simulink model "RefModel_TaskOutput"  (R2015b)
settings: configuration reference "CenterOutReachConfigSet" (kept outside this file)
undefined symbols (not defined in the file or in its folder): SimulinkParameter_TunableNote
settings Model: Creator=djoshea  LastModifiedBy=shenoylab
settings ConfigSetRef: SourceLocation=Base Workspace

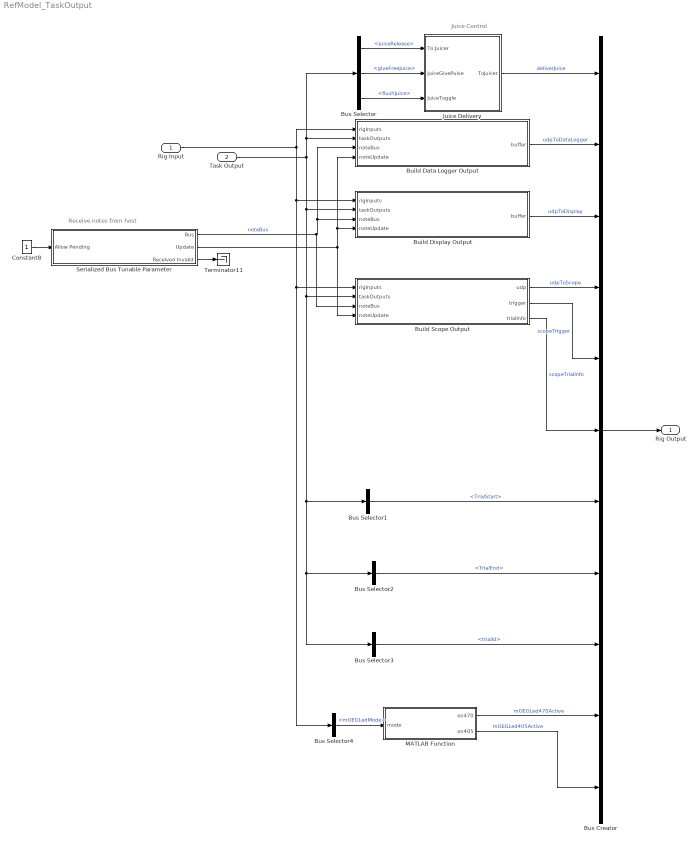
== system RefModel_TaskOutput ==
  note: Juice Control
  note: Receive notes from host
  Rig Input : Inport  OutDataTypeStr=Bus: RigInputBus  PortDimensions=1  SampleTime=[0.001,0]  Interpolate=off  BusOutputAsStruct=on
  Task Output : Inport  Port=2  OutDataTypeStr=Bus: TaskOutputBus  PortDimensions=1  SampleTime=[0.001,0]  Interpolate=off  BusOutputAsStruct=on
  Build Data Logger Output : MATLAB Function  TreatAsAtomicUnit=on
  Build Display Output : MATLAB Function  TreatAsAtomicUnit=on
  Build Scope Output : MATLAB Function  TreatAsAtomicUnit=on
  Bus Creator : BusCreator  Inputs=11  OutDataTypeStr=Bus: RigOutputBus  NonVirtualBus=on
  Bus Selector : BusSelector  OutputSignals=juiceRelease,taskControl.giveFreeJuice,taskControl.flushJuice
  Bus Selector1 : BusSelector  OutputSignals=TrialStart
  Bus Selector2 : BusSelector  OutputSignals=TrialEnd
  Bus Selector3 : BusSelector  OutputSignals=trialId
  Bus Selector4 : BusSelector  OutputSignals=scopeState.mOEGLedMode
  Constant8 : Constant  OutDataTypeStr=uint8
  Juice Delivery : Subsystem
  MATLAB Function : MATLAB Function  TreatAsAtomicUnit=on
  Serialized Bus Tunable Parameter : Subsystem  AncestorBlock=libBusSerialize/Serialized Bus Tunable Parameter  mask(BusSerialize Tunable Parameter Block){paramName='TunableNote'}
      mask prompts: paramName "Parameter Name"
      mask help: This block provides the value of a tunable Simulink.Parameter into the model. Since tunable parameters with xPC target can only be doubles, the functions BusSerialize.createTunableParameter and BusSerialize.setTunableParameter automatically handle typecasting and update counter insertion, and this block handles update detection, typecasting, and reshaping back to the original form. Currently, variable size parameters are not supported.
      mask init:
      | BusSerialize.maskSerializedBusTunableParameterBlockUpdate(gcb);
      mask Display:
      | port_label('output', 1, paramName);
      | port_label('output', 2, 'Update');
      | port_label('output', 3, 'Received Invalid');
      | port_label('input', 1, 'Allow Pending');
  Terminator11 : Terminator
  Rig Output : Outport  OutDataTypeStr=Bus: RigOutputBus  PortDimensions=1  SampleTime=[0.001,0]  BusOutputAsStruct=on
  wires:
  Rig Input/1 -> Bus Selector4/1, Build Scope Output/1(rigInputs), Build Display Output/1(rigInputs), Build Data Logger Output/1(rigInputs)
  Bus Creator/1 -> Rig Output/1
  Build Data Logger Output/1(buffer) -> Bus Creator/2  "udpToDataLogger"
  Build Display Output/1(buffer) -> Bus Creator/3  "udpToDisplay"
  Bus Selector/2 -> Juice Delivery/2(JuiceGivePulse)  "<giveFreeJuice>"
  Bus Selector/1 -> Juice Delivery/1(To Juicer)  "<juiceRelease>"
  Bus Selector/3 -> Juice Delivery/3(JuiceToggle)  "<flushJuice>"
  Juice Delivery/1(ToJuicer) -> Bus Creator/1  "deliverJuice"
  Constant8/1 -> Serialized Bus Tunable Parameter/1(Allow Pending)
  Serialized Bus Tunable Parameter/3(Received Invalid) -> Terminator11/1
  Serialized Bus Tunable Parameter/1(Bus) -> Build Scope Output/3(noteBus), Build Data Logger Output/3(noteBus), Build Display Output/3(noteBus)  "noteBus"
  Bus Selector1/1 -> Bus Creator/7  "<TrialStart>"
  Serialized Bus Tunable Parameter/2(Update) -> Build Scope Output/4(noteUpdate), Build Data Logger Output/4(noteUpdate), Build Display Output/4(noteUpdate)
  Build Scope Output/1(udp) -> Bus Creator/4  "udpToScope"
  Build Scope Output/2(trigger) -> Bus Creator/5  "scopeTrigger"
  Bus Selector2/1 -> Bus Creator/8  "<TrialEnd>"
  Build Scope Output/3(trialInfo) -> Bus Creator/6  "scopeTrialInfo"
  Task Output/1 -> Build Data Logger Output/2(taskOutputs), Bus Selector/1, Bus Selector3/1, Bus Selector2/1, Bus Selector1/1, Build Scope Output/2(taskOutputs), Build Display Output/2(taskOutputs)
  Bus Selector3/1 -> Bus Creator/9  "<trialId>"
  Bus Selector4/1 -> MATLAB Function/1(mode)  "<mOEGLedMode>"
  MATLAB Function/2(on405) -> Bus Creator/11  "mOEGLed405Active"
  MATLAB Function/1(on470) -> Bus Creator/10  "mOEGLed470Active"

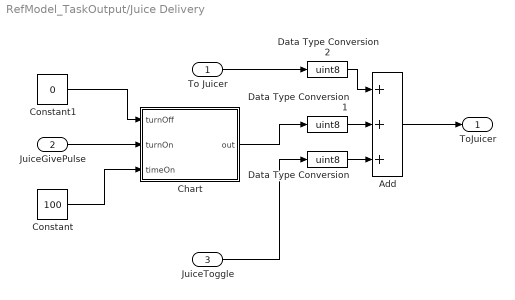
== system RefModel_TaskOutput/Juice Delivery ==
  To Juicer : Inport
  JuiceGivePulse : Inport  Port=2
  JuiceToggle : Inport  Port=3
  Add : Sum  Inputs=+++
  Chart : Stateflow chart  TreatAsAtomicUnit=on
  Constant : Constant  Value=100  OutDataTypeStr=uint32
  Constant1 : Constant  Value=0  OutDataTypeStr=uint8
  Data Type Conversion : DataTypeConversion  OutDataTypeStr=uint8
  Data Type Conversion1 : DataTypeConversion  OutDataTypeStr=uint8
  Data Type Conversion2 : DataTypeConversion  OutDataTypeStr=uint8
  ToJuicer : Outport
  wires:
  Data Type Conversion2/1 -> Add/1
  Data Type Conversion1/1 -> Add/2
  Data Type Conversion/1 -> Add/3
  Constant1/1 -> Chart/1(turnOff)
  JuiceToggle/1 -> Data Type Conversion/1
  Add/1 -> ToJuicer/1
  Constant/1 -> Chart/3(timeOn)
  JuiceGivePulse/1 -> Chart/2(turnOn)
  Chart/1(out) -> Data Type Conversion1/1
  To Juicer/1 -> Data Type Conversion2/1

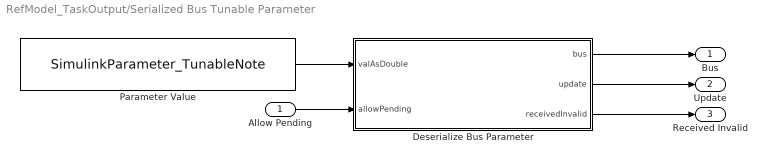
== system RefModel_TaskOutput/Serialized Bus Tunable Parameter ==
  Allow Pending : Inport
  Deserialize Bus Parameter : MATLAB Function  TreatAsAtomicUnit=on
  Parameter Value : Constant  Value=SimulinkParameter_TunableNote  OutDataTypeStr=double
  Bus : Outport  PortDimensions=1
  Update : Outport  Port=2  OutDataTypeStr=uint8  PortDimensions=1
  Received Invalid : Outport  Port=3  OutDataTypeStr=uint8  PortDimensions=1
  wires:
  Parameter Value/1 -> Deserialize Bus Parameter/1(valAsDouble)
  Allow Pending/1 -> Deserialize Bus Parameter/2(allowPending)
  Deserialize Bus Parameter/3(receivedInvalid) -> Received Invalid/1
  Deserialize Bus Parameter/1(bus) -> Bus/1
  Deserialize Bus Parameter/2(update) -> Update/1

== matlab function RefModel_TaskOutput/Build Scope Output ==
  data: udp output uint8 size=RigInfo.outputSizes.udpToScope; rigInputs input Bus: RigInputBus size=1; taskOutputs input Bus: TaskOutputBus size=1; noteBus input Bus: NoteBus size=1; noteUpdate input uint8 size=1; RigInfo parameter size=1; trigger output uint8 size=1; trialInfo output uint8 size=RigInfo.outputSizes.trialInfoToScope
function [udp, trigger, trialInfo] = buildScopeOutput(rigInputs, taskOutputs, noteBus, noteUpdate, RigInfo)
%#codegen

    coder.cinclude('<stdlib.h>'); % for sprintf

    coder.varsize('udp', RigInfo.outputSizes.udpToScope);
    coder.varsize('trialInfo', RigInfo.outputSizes.trialInfoToScope);
    
    bEmpty = zeros(0, 1, 'uint8');
    
    
    

    %initialize persistant variables
    persistent pTrialId;
    if isempty(pTrialId)
        pTrialId = uint32(0);
    end
    
    persistent pConditionId;
    if isempty(pConditionId)
        pConditionId = uint16(0);
    end
    
    persistent pConditionsToDecode;
    if isempty(pConditionsToDecode)
        pConditionsToDecode = uint8(zeros(4,1));
    end
    
    persistent pUseNextFrame;
    if isempty(pUseNextFrame)
        pUseNextFrame = uint8(0);
    end
    
    persistent pImageDecoderTraining;
    if isempty(pImageDecoderTraining)
        pImageDecoderTraining = uint8(0);
    end
    
    persistent pResetDecoder;
    if isempty(pResetDecoder)
        pResetDecoder = uint8(0);
    end
    
    persistent pSaveTag;
    if isempty(pSaveTag)
        pSaveTag = uint32(0);
    end
    
    % detect if any of these have changed and update persistent variable
    doBytePack = false;
    if (taskOutputs.trialId ~= pTrialId)    
        doBytePack = true;
        pTrialId = uint32(taskOutputs.trialId);
    end
    
    if (taskOutputs.condition.conditionId ~= pConditionId)
        doBytePack = true;
        pConditionId = uint16(taskOutputs.condition.conditionId);
    end
    
    if all(taskOutputs.param.conditionsToDecode ~= pConditionsToDecode)
        doBytePack = true;
        pConditionsToDecode = uint8(taskOutputs.param.conditionsToDecode);
    end
    
    if (taskOutputs.trialData.useNextFrame ~= pUseNextFrame)
        doBytePack = true;
        pUseNextFrame = uint8(taskOutputs.trialData.useNextFrame);
    end
    
    if (taskOutputs.param.imageDecoderTraining ~= pImageDecoderTraining)
        doBytePack = true;
        pImageDecoderTraining = uint8(taskOutputs.param.imageDecoderTraining);
    end
    
    if (taskOutputs.param.resetImageDecoder ~= pResetDecoder)
        doBytePack = true;
        pResetDecoder = uint8(taskOutputs.param.resetImageDecoder);
    end
    
    if (taskOutputs.dataLoggerInfo.saveTag ~= pSaveTag)
        doBytePack = true;
        pSaveTag = uint32(taskOutputs.dataLoggerInfo.saveTag);
    end
    
    % Do the byte packing if anything has updated
    if doBytePack
        bHeader = uint8('#D')';
        bTrialId = typecast(taskOutputs.trialId,'uint8')';
        bConditionId = typecast(taskOutputs.condition.conditionId,'uint8')';
        bConditionsToDecode = uint8(taskOutputs.param.conditionsToDecode);  % already a logical
        bUseNextFrame = typecast(taskOutputs.trialData.useNextFrame,'uint8')';
        bImageDecoderTraining = typecast(taskOutputs.param.imageDecoderTraining,'uint8')';
        bResetDecoder = typecast(taskOutputs.param.resetImageDecoder,'uint8')';
        bSaveTag = typecast(pSaveTag, 'uint8')';
        udp = [bHeader; bTrialId; bConditionId; bConditionsToDecode; ...
            bUseNextFrame; bImageDecoderTraining; bResetDecoder; bSaveTag];
        trigger = uint8(1);
    else
        trigger = uint8(0);
        udp = bEmpty;
    end
    
    if ~isempty(udp)
        % add null-terminator for udp and make sure byte count is even,
        % needed for Windows, not sure why
        if mod(numel(udp), 2) == 0
            udp = [udp; uint8(' '); uint8(0)];
        else
            udp = [udp; uint8(0)];
        end
    end
    
     maxNextTrial = 500;
     trialInfo = bEmpty;

    % serialize scope commands
    if taskOutputs.taskControl.controlImaging && ~isempty(taskOutputs.scopeCommandQueue)
        % loop through scope commands and generate the command text for
        % each 
        coder.varsize('bNextTrial', maxNextTrial);
        for i = 1:numel(taskOutputs.scopeCommandQueue)
            command = taskOutputs.scopeCommandQueue(i);
            
            switch command
                case ScopeCommand.NextTrial
                   % also generate a command to send to the PrairieView
                    % voltage recording
                    nBytes = int32(0);
                    trialInfoBuffer = zeros(RigInfo.outputSizes.trialInfoToScope, 1, 'uint8');
                    nBytes = coder.ceval('sprintf', coder.ref(trialInfoBuffer), ...
                        ['id=%d,c=%d,d=' enumToString_DirectionName(taskOutputs.condition.targetDirectionName)' ';' uint8(0)], ...
                        taskOutputs.trialId, taskOutputs.condition.conditionId);
                     if nBytes > RigInfo.outputSizes.trialInfoToScope
                         trialInfo = trialInfoBuffer(1:RigInfo.outputSizes.trialInfoToScope);
                     else
                         trialInfo = trialInfoBuffer(1:nBytes);
                     end
            end
        end
    end
    
    
    
    
end

== matlab function RefModel_TaskOutput/MATLAB Function ==
  data: mode input Enum: LedMode size=1; on470 output uint8 size=1; on405 output uint8 size=1
function [on470, on405] = getLedStatus(mode)
%#codegen

    on470 = uint8(0);
    on405 = uint8(0);
    
    switch mode
        case LedMode.Off
            
        case LedMode.CW405
            on405 = uint8(1);

        case LedMode.CW470
            on470 = uint8(1);
    
        case LedMode.Alternating405_470
            on470 = uint8(1);
            on405 = uint8(1);
    end
end

== stateflow chart RefModel_TaskOutput/Juice Delivery/Chart ==
  state On
    en:
    out = uint8(1);
    ex:
    out = uint8(0);
  state Waiting
  (default) -> Waiting
  Waiting -> On : [turnOn==1]
  On -> Waiting [order 1] : after(timeOn, tick)
  On -> Waiting [order 2] : [turnOff==1]
  data: turnOff input uint8 size=1; turnOn input uint8 size=1; timeOn input uint32 size=1; out output uint8 size=1

== matlab function RefModel_TaskOutput/Serialized Bus Tunable Parameter/Deserialize Bus Parameter ==
  data: valAsDouble input double; bus output Bus: NoteBus size=1; update output uint8 size=1; allowPending input uint8 size=1; receivedInvalid output uint8 size=1
function [bus, update, receivedInvalid] = deserializeBusParameter(valAsDouble, allowPending)
%#codegen

    % typecast to bytes
    valAsBytes = typecast(valAsDouble, 'uint8');

    % use the first byte as updateCounter, check for whether counter has been incremented
    thisCounter = valAsBytes(1);
    persistent pLastCounter;
    if isempty(pLastCounter)
        pLastCounter = thisCounter;
    end
    if pLastCounter ~= thisCounter
        recvUpdate = uint8(1);
        pLastCounter = thisCounter;
    else
        recvUpdate = uint8(0);
    end
    startOffset = 2;

    % external cached output for when allowPending 
    persistent pBusOut;
    if isempty(pBusOut)
        pBusOut = initializeBus_NoteBus();
    end

    % parse incoming bytes if allowing updates
    receivedInvalid = uint8(0);
    if allowPending
        [bus, valid] = deserializeBus_NoteBus(valAsBytes, startOffset);
        if valid
            % update internal cache
            pBusOut = bus;
        else
            % don't update internal cache, output internal cache
            bus = pBusOut;
            receivedInvalid = uint8(1);
            recvUpdate = uint8(0);
        end
    else
        bus = pBusOut;
    end

    % track whether we have a pending update
    persistent pPending;
    if isempty(pPending), pPending = uint8(0); end
    if recvUpdate
        if allowPending
            % update goes out immediately
            update = uint8(1);
            pPending = uint8(0);
        else
            % queue pending update
            update = uint8(0);
            pPending = uint8(1);
        end
    else
        if allowPending
            % release pending
            update = pPending;
            pPending = uint8(0);
        else
            % do nothing
            update = uint8(0);
        end
    end

    % reset fields marked with .resetImmediately immediately after update
    if ~update

    end
end

== matlab function RefModel_TaskOutput/Build Data Logger Output ==
  data: buffer output uint8 size=RigInfo.outputSizes.udpToDataLogger; rigInputs input; taskOutputs input; noteBus input Bus: NoteBus size=1; noteUpdate input uint8 size=1; RigInfo parameter
function buffer = buildDataLoggerOutput(rigInputs, taskOutputs, noteBus, noteUpdate, RigInfo)
%#codegen

bEmpty = zeros(0, 1, 'uint8');
coder.varsize('buffer', RigInfo.outputSizes.udpToDataLogger);
buffer = zeros(0, 1, 'uint8');

if taskOutputs.taskControl.saveData && taskOutputs.taskControl.runTask && ~taskOutputs.trialData.inPurgatory

    % timestamp for data logger
    timestamp = rigInputs.clock;

    % send TrialStart info
    if taskOutputs.TrialStart
        % send data logger info
        bDataInfo = serializeBusWithDataLoggerHeader_DataLoggerInfoBus(...
            taskOutputs.dataLoggerInfo, BusSerialize.GroupTypes.Control, uint8('info'), timestamp);

        % send next trial with new trial id
        % once TrialStart goes high, the trialId field has already updated
        nextTrialBus = initializeBus_DataLoggerNextTrialBus();
        nextTrialBus.nextTrial = taskOutputs.trialId;
        bNextTrial = serializeBusWithDataLoggerHeader_DataLoggerNextTrialBus(...
            nextTrialBus, BusSerialize.GroupTypes.Control, uint8('nextTrial'), timestamp);

        % send this trial's parameters
        bParam = serializeBusWithDataLoggerHeader_ParamBus(...
            taskOutputs.param, BusSerialize.GroupTypes.Parameter, uint8('param'), timestamp);

        % send this trial's condition
        bCondition = serializeBusWithDataLoggerHeader_ConditionBus(...
            taskOutputs.condition, BusSerialize.GroupTypes.Parameter, uint8('condition'), timestamp);
    else
        bDataInfo = bEmpty;
        bNextTrial = bEmpty;
        bParam = bEmpty;
        bCondition = bEmpty;
    end
    
    if taskOutputs.TrialITI
        % send TrialDataOutputBus
        bTrialData = serializeBusWithDataLoggerHeader_TrialDataOutputBus(...
            taskOutputs.trialDataOutput, BusSerialize.GroupTypes.Parameter, uint8('trialData'), timestamp);
        
        % send MicroscopeStateBus
        bScopeState = serializeBusWithDataLoggerHeader_MicroscopeStateBus(...
            rigInputs.scopeState, BusSerialize.GroupTypes.Parameter, uint8('scope'), timestamp);
    else
        bTrialData = bEmpty;
        bScopeState = bEmpty;
    end

    % serialize handOutput on handUpdate
    if rigInputs.hand.handUpdate
        bHand = serializeBusWithDataLoggerHeader_HandOutputBus(...
            taskOutputs.handOutput, BusSerialize.GroupTypes.Analog, uint8('hand'), timestamp);
    else
        bHand = bEmpty;
    end
    
    % serialize eyeOutput on eyeUpdate
    if rigInputs.eye.eyeUpdate
        bEye = serializeBusWithDataLoggerHeader_EyeOutputBus(...
            taskOutputs.eyeOutput, BusSerialize.GroupTypes.Analog, uint8('eye'), timestamp);
    else
        bEye = bEmpty;
    end
    
    % serialize analogOutput (every tick)
    bAnalog = serializeBusWithDataLoggerHeader_AnalogOutputBus(...
            taskOutputs.analogOutput, BusSerialize.GroupTypes.Analog, uint8('analog'), timestamp);
        
    % serialize scopeTiming (every tick)
    bScopeTiming = serializeBusWithDataLoggerHeader_ScopeTimingBus(...
            rigInputs.scopeTiming, BusSerialize.GroupTypes.Analog, uint8('scopeTiming'), timestamp);
    
    % serialize mOEGFrameInfo (every tick)
    bmOEGFrameInfo = serializeBusWithDataLoggerHeader_mOEGFrameInfoBus(...
            rigInputs.mOEGFrameInfo, BusSerialize.GroupTypes.Analog, uint8('mOEGFrameInfo'), timestamp);
        
    if rigInputs.decoderBus.decoderUpdate
        bDecoderInfo = serializeBusWithDataLoggerHeader_DecoderBus(...
                rigInputs.decoderBus, BusSerialize.GroupTypes.Analog, uint8('decoderInfo'), timestamp);
    else
        bDecoderInfo = bEmpty;
    end
        
    % serialize scope events
    coder.varsize('bScopeEvents', 1000, 1);
    bScopeEvents = bEmpty;
    scopeEventBus = initializeBus_ScopeEventBus();
    if rigInputs.scopeTiming.cameraFrameEnd
        scopeEventBus.event = ScopeEvent.CameraFrameEnd;
        bScopeEvents = [bScopeEvents; serializeBusWithDataLoggerHeader_ScopeEventBus(...
            scopeEventBus, BusSerialize.GroupTypes.Event, uint8('scopeEvent'), timestamp)];
    end
        
    % serialize noteBus on update
    if noteUpdate
        bNote = serializeBusWithDataLoggerHeader_NoteBus(...
            noteBus, BusSerialize.GroupTypes.Note, uint8('note'), timestamp);
    else
        bNote = bEmpty;
    end

    % serialize TaskEvents
    coder.varsize('bTaskEvents', 1000, 1);
    bTaskEvents = bEmpty;
    eventBus = initializeBus_TaskEventBus();
    for i = 1:numel(taskOutputs.taskEventQueue)
        eventBus.event = taskOutputs.taskEventQueue(i);
        bTaskEvents = [bTaskEvents; serializeBusWithDataLoggerHeader_TaskEventBus(...
            eventBus, BusSerialize.GroupTypes.Event, uint8('taskEvent'), timestamp)]; %#ok<AGROW>
        
        coder.ceval('printf', ['TaskEvent ' enumToString_TaskEvent(eventBus.event) '; ' uint8([10 0])]);
    end

    buffer = [bDataInfo; bNextTrial; bCondition; bTrialData; bTaskEvents; bParam; bScopeState; ...
        bHand; bEye; bAnalog; bScopeTiming; bScopeEvents; bmOEGFrameInfo; bDecoderInfo; bNote];
    
    if ~isempty(buffer)
        % add null-terminator for udp and make sure byte count is even,
        % needed for Windows, not sure why
        if mod(numel(buffer), 2) ~= 0
            buffer = [buffer; uint8(0)];
        end
    end
end

end

== matlab function RefModel_TaskOutput/Build Display Output ==
  data: buffer output uint8 size=RigInfo.outputSizes.udpToDisplay; rigInputs input; taskOutputs input; noteBus input Bus: NoteBus size=1; noteUpdate input uint8 size=1; RigInfo parameter
function buffer = buildDisplayOutput(rigInputs, taskOutputs, noteBus, noteUpdate, RigInfo)
%#codegen

    coder.varsize('buffer', RigInfo.outputSizes.udpToDisplay);
    bEmpty = zeros(0, 1, 'uint8');

    % timestamp for data logger
    timestamp = rigInputs.clock;

    % send TrialStart info
    if taskOutputs.TrialStart
        % send data logger info
        bDataInfo = serializeBusWithDataLoggerHeader_DataLoggerInfoBus(...
            taskOutputs.dataLoggerInfo, BusSerialize.GroupTypes.Control, uint8('info'), timestamp);

        % send next trial with new trial id
        nextTrialBus = initializeBus_DataLoggerNextTrialBus();
        nextTrialBus.nextTrial = taskOutputs.trialId;
        bNextTrial = serializeBusWithDataLoggerHeader_DataLoggerNextTrialBus(...
            nextTrialBus, BusSerialize.GroupTypes.Control, uint8('nextTrial'), timestamp);

        % send this trial's parameters
        bParam = serializeBusWithDataLoggerHeader_ParamBus(...
            taskOutputs.param, BusSerialize.GroupTypes.Parameter, uint8('P'), timestamp);

        % send this trial's condition
        bCondition = serializeBusWithDataLoggerHeader_ConditionBus(...
            taskOutputs.condition, BusSerialize.GroupTypes.Parameter, uint8('C'), timestamp);

        % set display task
        busSetTask = initializeBus_DisplaySetTaskBus();
        busSetTask.taskName = uint8('CenterOutReachTask');
        busSetTask.taskVersion = uint32(20150121);
        bSetTask = serializeBusWithDataLoggerHeader_DisplaySetTaskBus(...
            busSetTask, BusSerialize.GroupTypes.Parameter, uint8('setTask'), timestamp);
    else
        bDataInfo = bEmpty;
        bNextTrial = bEmpty;
        bParam = bEmpty;
        bCondition = bEmpty;
        bSetTask = bEmpty;
    end

    % serialize task commands
    if ~isempty(taskOutputs.displayCommandQueue)
        coder.varsize('bCommand', 10000);
        % send trialData before each group of taskCommands
        bCommand = serializeBusWithDataLoggerHeader_TrialDataBus(...
            taskOutputs.trialData, BusSerialize.GroupTypes.Parameter, uint8('trialData'), timestamp);

        % loop through task commands and serialize them, crucial that this
        % be analog
        commandBus = initializeBus_DisplayCommandBus();
        for i = 1:numel(taskOutputs.displayCommandQueue)
            commandBus.taskCommand = taskOutputs.displayCommandQueue(i);
            bCommand = [bCommand; serializeBusWithDataLoggerHeader_DisplayCommandBus(...
                commandBus, BusSerialize.GroupTypes.Analog, uint8('taskCommand'), timestamp)]; %#ok<AGROW>
        end
    else
        bCommand = bEmpty;
    end

    % serialize handOutput if updated as Param
    if rigInputs.hand.handUpdate
        bHand = serializeBusWithDataLoggerHeader_HandOutputBus(...
            taskOutputs.handOutput, BusSerialize.GroupTypes.Parameter, uint8('handInfo'), timestamp);
    else
        bHand = bEmpty;
    end

    % serialize noteBus on update
    if noteUpdate
        bNote = serializeBusWithDataLoggerHeader_NoteBus(...
            noteBus, BusSerialize.GroupTypes.Note, uint8('note'), timestamp);
    else
        bNote = bEmpty;
    end

    % assemble the final output
    buffer = [bDataInfo; bNextTrial; bParam; bCondition; bSetTask; bCommand; bHand; bNote];

end
